simulink model "main"  (R2022b)
settings: Solver=FixedStepDiscrete  StartTime=0.0  StopTime=10.0  FixedStep=0.005  RelTol=1e-3
libraries: arduinolib x1
settings Model: ExtModeTrigDuration=2  Creator=F64236C  LastModifiedBy=F64236C
settings OptimizationCC: EnhancedBackFolding=on  PassReuseOutputArgsAs=Individual arguments  ZeroExternalMemoryAtStartup=off  ZeroInternalMemoryAtStartup=off  MaxStackSize=64  OptimizeBlockOrder=speed  DifferentSizesBufferReuse=on  OptimizationCustomize=off  EfficientTunableParamExpr=on
settings DebuggingCC: ParameterTunabilityLossMsg=error
settings HardwareCC: ProdBitPerInt=16  ProdBitPerPointer=16  ProdBitPerSizeT=16  ProdBitPerPtrDiffT=16  ProdLargestAtomicFloat=None  ProdWordSize=8  ProdHWDeviceType=Atmel->AVR
settings SFSimCC: MATLABDynamicMemAlloc=off
settings RTWCC: Description=Embedded Coder  SystemTargetFile=ert.tlc  HardwareBoard=Arduino Uno  TLCOptions=-aInlineSetEventsForThisBaseRateFcn=TLC_FALSE -aSuppressMultiTaskScheduler=TLC_FALSE -aRateBasedStepFcn=1  TemplateMakefile=ert_default_tmf  Toolchain=Arduino AVR
settings CodeAppCC: ForceParamTrailComments=on  IgnoreCustomStorageClasses=off  OperatorAnnotations=on  SimulinkDataObjDesc=on  SFDataObjDesc=on  InsertBlockDesc=on
settings ERTTargetCC: SupportContinuousTime=on  SupportVariableSizeSignals=on  ExtModeTransport=3  ExtModeStaticAlloc=on  ExtModeAutomaticAllocSize=off  ExtModeStaticAllocSize=250  ExtModeMexFile=ext_xcp  ExtModeIntrfLevel=Level2 - Open

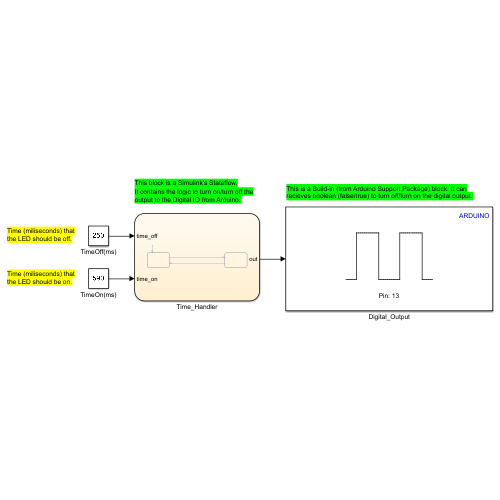
[thumbnail: Simulink's stored preview of the top-level diagram]
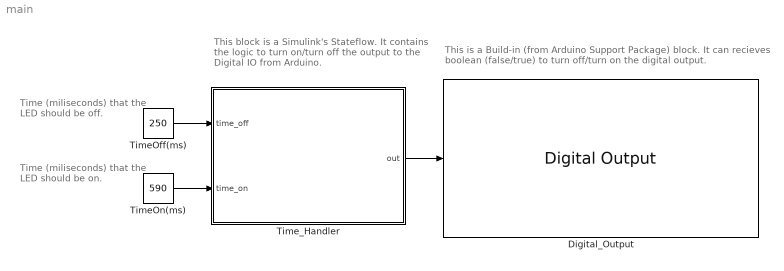
== system main ==
  note: Time (miliseconds) that the LED should be off.
  note: This block is a Simulink's Stateflow.
      | It contains the logic to turn on/turn off the output to the Digital IO from Arduino.
  note: This is a Build-in (from Arduino Support Package) block. It can recieves boolean (false/true) to turn off/turn on the digital output.
  note: Time (miliseconds) that the LED should be on.
  Digital_Output : arduinolib/Digital Output  pinNumber=13  Direction=output  blockPlatform=arduino
  TimeOff(ms) : Constant  Value=250  OutDataTypeStr=uint32
  TimeOn(ms) : Constant  Value=590  OutDataTypeStr=uint32
  Time_Handler : Stateflow chart  TreatAsAtomicUnit=on
  wires:
  Time_Handler/1(out) -> Digital_Output/1
  TimeOff(ms)/1 -> Time_Handler/1(time_off)
  TimeOn(ms)/1 -> Time_Handler/2(time_on)

== stateflow chart main/Time_Handler ==
  state on
    en:
    out = true;
  state off
    en:
    out = false;
  (default) -> on
  on -> off : [after(time_on,msec)]
  off -> on : [after(time_off,msec)]
  data: time_off input uint32; time_on input uint32; out output boolean
